simulink model "Controlador_PI"  (R2021a)
settings: Solver=VariableStepAuto  StartTime=0.0  StopTime=2  RelTol=1e-3
libraries: cstblocks x4
settings Model: Creator=sofia  LastModifiedBy=sofia

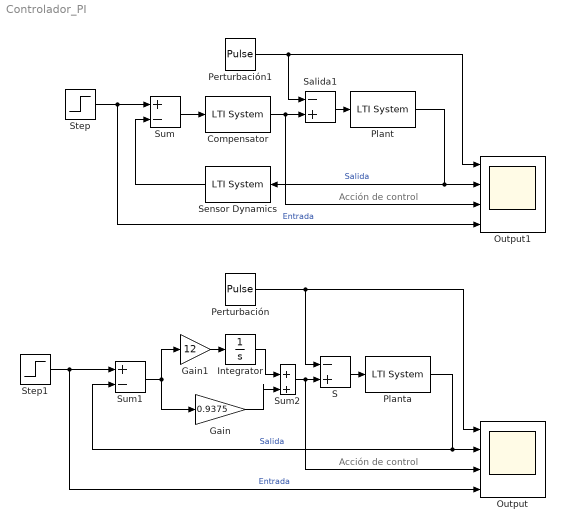
== system Controlador_PI ==
  note: Acción de control
  note: Acción de control
  Compensator : cstblocks/LTI System  sys=C  IC=[]
  Gain : Gain  Gain=0.9375
  Gain1 : Gain  Gain=12
  Integrator : Integrator
  Output : Scope  NumInputPorts=4
  Output1 : Scope  NumInputPorts=4
  Perturbación : DiscretePulseGenerator  PulseType=Time based  PulseWidth=25  PhaseDelay=0.7
  Perturbación1 : DiscretePulseGenerator  PulseType=Time based  PulseWidth=25  PhaseDelay=0.7
  Plant : cstblocks/LTI System  sys=G  IC=[]
  Planta : cstblocks/LTI System  sys=G  IC=[]
  S : Sum  Inputs=-+
  Salida1 : Sum  Inputs=-+
  Sensor Dynamics : cstblocks/LTI System  sys=H  IC=[]
  Step : Step  Tag=Entrada  Time=0.1  After=4  SampleTime=0
  Step1 : Step  Tag=Entrada  Time=0.1  After=4  SampleTime=0
  Sum : Sum  Inputs=+-
  Sum1 : Sum  Inputs=+-
  Sum2 : Sum  Inputs=|+|+|
  wires:
  Step/1 -> Output1/4, Sum/1  "Entrada"
  Sensor Dynamics/1 -> Sum/2
  Sum/1 -> Compensator/1
  Compensator/1 -> Output1/3, Salida1/2
  Plant/1 -> Output1/2, Sensor Dynamics/1  "Salida"
  Step1/1 -> Sum1/1, Output/4  "Entrada"
  Planta/1 -> Sum1/2, Output/2  "Salida"
  Gain1/1 -> Integrator/1
  Sum2/1 -> S/2, Output/3
  Integrator/1 -> Sum2/1
  Gain/1 -> Sum2/2
  Sum1/1 -> Gain1/1, Gain/1
  Perturbación1/1 -> Output1/1, Salida1/1
  Salida1/1 -> Plant/1
  Perturbación/1 -> S/1, Output/1
  S/1 -> Planta/1
